simulink model "OsciladorVanDerPol"  (R2021a)
settings: Solver=ode15s  StartTime=0.0  StopTime=10000  RelTol=1e-3
settings Model: Creator=Aula  LastModifiedBy=Aula

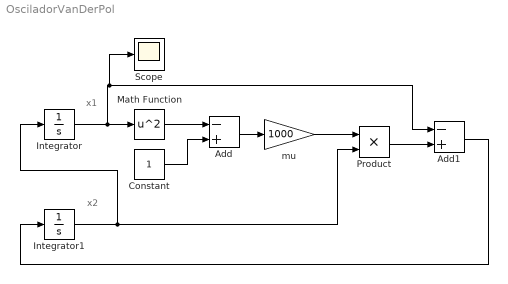
== system OsciladorVanDerPol ==
  note: x2
  note: x1
  Add : Sum  Inputs=-+
  Add1 : Sum  Inputs=-+
  Constant : Constant
  Integrator : Integrator  InitialCondition=2
  Integrator1 : Integrator
  Math Function : Math  Operator=square  SaturateOnIntegerOverflow=on
  Product : Product
  Scope : Scope
  mu : Gain  Gain=1000
  wires:
  Integrator/1 -> Scope/1, Add1/1, Math Function/1
  Math Function/1 -> Add/1
  Constant/1 -> Add/2
  Add/1 -> mu/1
  mu/1 -> Product/1
  Integrator1/1 -> Integrator/1, Product/2
  Product/1 -> Add1/2
  Add1/1 -> Integrator1/1
